simulink model "Problem_1"  (R2020a)
settings: Solver=VariableStepAuto  StartTime=0.0  StopTime=10.0  RelTol=1e-3
settings Model: Creator=Saqlain  LastModifiedBy=Saqlain

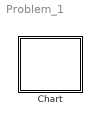
== system Problem_1 ==
  Chart : Stateflow chart  TreatAsAtomicUnit=on

== stateflow chart Problem_1/Chart ==
  state got_0
  state got_nickel
  state got_dime
  (default) -> got_0
  got_0 -> got_nickel [order 1] : [coin == 1]{soda = 0}
  got_0 -> got_dime [order 2] : [coin == 2]{soda = 0}
  got_nickel -> got_dime : [coin == 1]{soda = 0}
